simulink model "temp_change"  (R2024b)
settings: Solver=VariableStepAuto  StartTime=0.0  StopTime=10.0  RelTol=1e-3
settings Model: Creator=Thanu  LastModifiedBy=Thanu

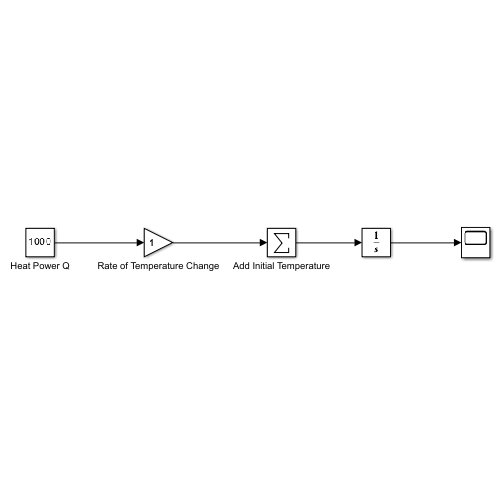
[thumbnail: Simulink's stored preview of the top-level diagram]
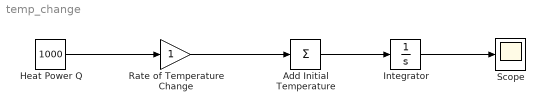
== system temp_change ==
  Add Initial Temperature : Sum  Inputs=+
  Heat Power Q : Constant  Value=1000
  Integrator : Integrator
  Rate of Temperature Change : Gain
  Scope : Scope
  wires:
  Heat Power Q/1 -> Rate of Temperature Change/1
  Integrator/1 -> Scope/1
  Rate of Temperature Change/1 -> Add Initial Temperature/1
  Add Initial Temperature/1 -> Integrator/1
